simulink model "MBSE_WindowsMIL"  (R2020b)
settings: Solver=VariableStepAuto  StartTime=0.0  StopTime=10.0  RelTol=1e-3
undefined symbols (not defined in the file): sigbuilder_block
libraries: simulink x8
settings Model: Creator=Training  LastModifiedBy=Training

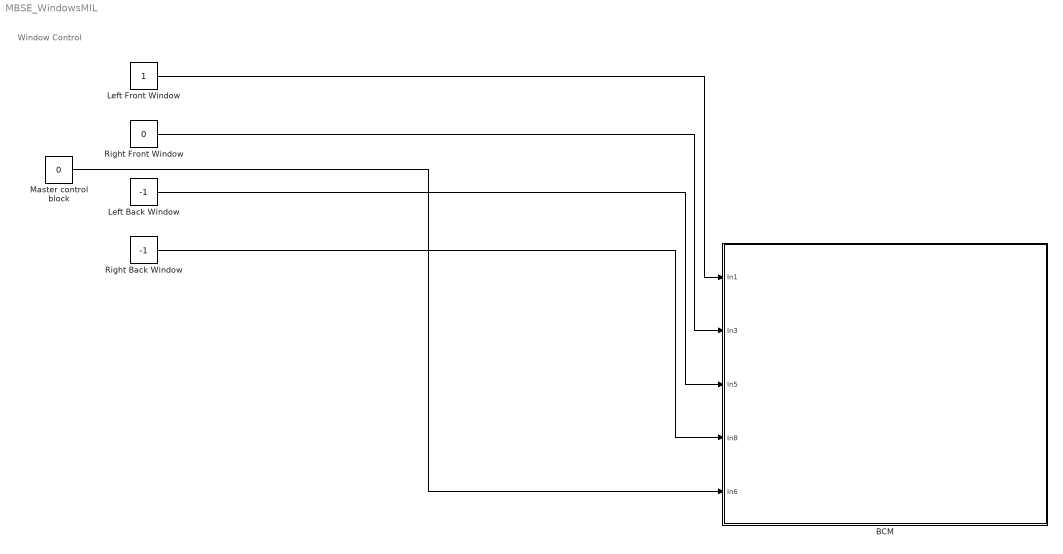
== system MBSE_WindowsMIL ==
  note: Window Control
  BCM : Subsystem
  Left Back Window : Constant  Value=-1
  Left Front Window : Constant
  Master control block : Constant  Value=0
  Right Back Window : Constant  Value=-1
  Right Front Window : Constant  Value=0
  wires:
  Master control block/1 -> BCM/5(In6)
  Right Back Window/1 -> BCM/4(In8)
  Left Back Window/1 -> BCM/3(In5)
  Right Front Window/1 -> BCM/2(In3)
  Left Front Window/1 -> BCM/1(In1)

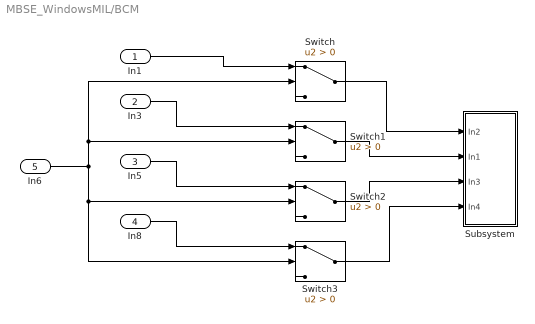
== system MBSE_WindowsMIL/BCM ==
  In1 : Inport
  In3 : Inport  Port=2
  In5 : Inport  Port=3
  In8 : Inport  Port=4
  In6 : Inport  Port=5
  Subsystem : Subsystem
  Switch{,1..3} (4 alike) : Switch  Criteria=u2 > Threshold
  wires:
  In8/1 -> Switch3/1
  In6/1 -> Switch/2, Switch1/2, Switch3/2, Switch2/2
  Switch/1 -> Subsystem/1(In2)
  In3/1 -> Switch1/1
  Switch1/1 -> Subsystem/2(In1)
  In5/1 -> Switch2/1
  Switch3/1 -> Subsystem/4(In4)
  Switch2/1 -> Subsystem/3(In3)
  In1/1 -> Switch/1

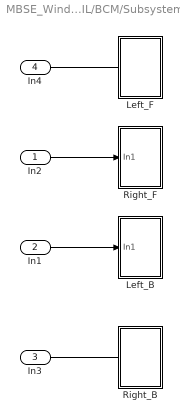
== system MBSE_WindowsMIL/BCM/Subsystem ==
  In2 : Inport
  In1 : Inport  Port=2
  In3 : Inport  Port=3
  In4 : Inport  Port=4
  Left_B : Subsystem
  Left_F : Subsystem
  Right_B : Subsystem
  Right_F : Subsystem
  wires:
  In4/1 -> ?
  In1/1 -> Left_B/1(In1)
  In2/1 -> Right_F/1(In1)
  In3/1 -> ?

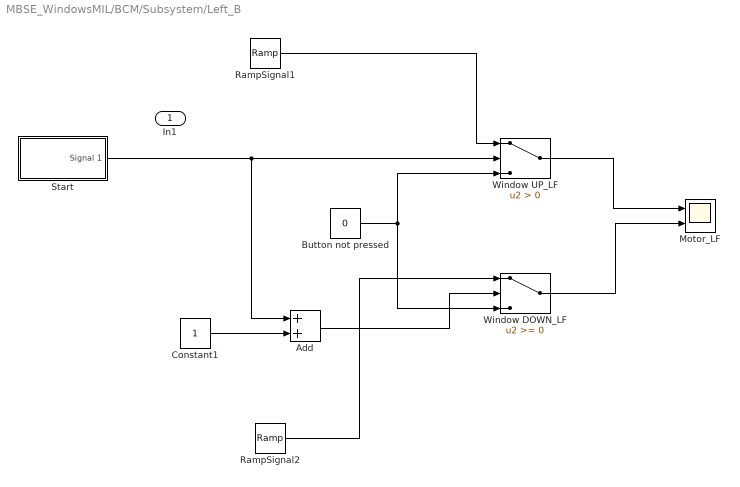
== system MBSE_WindowsMIL/BCM/Subsystem/Left_B ==
  In1 : Inport
  Add : Sum
  Button not pressed : Constant  Value=0
  Constant1 : Constant
  Motor_LF : Scope  NumInputPorts=2
  RampSignal1 : simulink/Sources/Ramp  slope=1  start=0  InitialOutput=0
  RampSignal2 : simulink/Sources/Ramp  slope=1  start=0  InitialOutput=0
  Start : Subsystem  Tag=STV Subsys  LoadFcn=sigbuilder_block('load');  StartFcn=sigbuilder_block('start');  StopFcn=sigbuilder_block('stop');  ClipboardFcn=sigbuilder_block('clipboard');  mask(Sigbuilder block){tuvar=[0:10]}
      mask help: Simulink:masks:SigbuilderBlock_MD
      mask init:
      | if ~strcmp(get_param(bdroot(gcbh),'SimulationStatus'),'stopped') tuvar = sigbuilder_block('maskInit'); end
      settings: CopyFcn=sigbuilder_block('copy');  DeleteFcn=sigbuilder_block('delete');  ModelCloseFcn=sigbuilder_block('modelClose');  PreSaveFcn=sigbuilder_block('preSave');  PauseFcn=sigbuilder_block('pause');  ContinueFcn=sigbuilder_block('continue');  NameChangeFcn=sigbuilder_block('namechange');  OpenFcn=sigbuilder_block('open',[437.6 199.2 550.4 400 ]);  CloseFcn=sigbuilder_block('close');
      mask Display: plot(0, 0, 100, 100,[2, 2, 32, 32, 2], [68, 8, 8, 68, 68],[32, 2], [38, 38], [32, 19, 2],[53, 60, 44], [32, 17, 17, 2],[16, 16, 31, 31]);txt = getActiveGroup(gcbh);text(2, 100, txt,'verticalAlignment', 'top');
  Window DOWN_LF : Switch
  Window UP_LF : Switch  Criteria=u2 > Threshold
  wires:
  Add/1 -> Window DOWN_LF/2
  Button not pressed/1 -> Window UP_LF/3, Window DOWN_LF/3
  Constant1/1 -> Add/2
  RampSignal2/1 -> Window DOWN_LF/1
  Window DOWN_LF/1 -> Motor_LF/2
  Start/1(Signal 1) -> Add/1, Window UP_LF/2
  RampSignal1/1 -> Window UP_LF/1
  Window UP_LF/1 -> Motor_LF/1

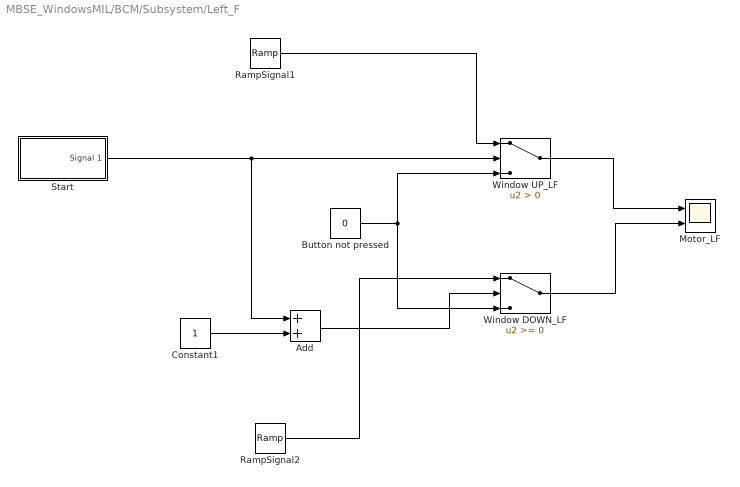
== system MBSE_WindowsMIL/BCM/Subsystem/Left_F ==
  Add : Sum
  Button not pressed : Constant  Value=0
  Constant1 : Constant
  Motor_LF : Scope  NumInputPorts=2
  RampSignal1 : simulink/Sources/Ramp  slope=1  start=0  InitialOutput=0
  RampSignal2 : simulink/Sources/Ramp  slope=1  start=0  InitialOutput=0
  Start : Subsystem  Tag=STV Subsys  LoadFcn=sigbuilder_block('load');  StartFcn=sigbuilder_block('start');  StopFcn=sigbuilder_block('stop');  ClipboardFcn=sigbuilder_block('clipboard');  mask(Sigbuilder block){tuvar=[0:10]}
      mask help: Simulink:masks:SigbuilderBlock_MD
      mask init:
      | if ~strcmp(get_param(bdroot(gcbh),'SimulationStatus'),'stopped') tuvar = sigbuilder_block('maskInit'); end
      settings: CopyFcn=sigbuilder_block('copy');  DeleteFcn=sigbuilder_block('delete');  ModelCloseFcn=sigbuilder_block('modelClose');  PreSaveFcn=sigbuilder_block('preSave');  PauseFcn=sigbuilder_block('pause');  ContinueFcn=sigbuilder_block('continue');  NameChangeFcn=sigbuilder_block('namechange');  OpenFcn=sigbuilder_block('open',[437.6 199.2 550.4 400 ]);  CloseFcn=sigbuilder_block('close');
      mask Display: plot(0, 0, 100, 100,[2, 2, 32, 32, 2], [68, 8, 8, 68, 68],[32, 2], [38, 38], [32, 19, 2],[53, 60, 44], [32, 17, 17, 2],[16, 16, 31, 31]);txt = getActiveGroup(gcbh);text(2, 100, txt,'verticalAlignment', 'top');
  Window DOWN_LF : Switch
  "Window UP_LF " : Switch  Criteria=u2 > Threshold
  wires:
  Add/1 -> Window DOWN_LF/2
  Button not pressed/1 -> "Window UP_LF "/3, Window DOWN_LF/3
  Constant1/1 -> Add/2
  RampSignal2/1 -> Window DOWN_LF/1
  Window DOWN_LF/1 -> Motor_LF/2
  Start/1(Signal 1) -> Add/1, "Window UP_LF "/2
  RampSignal1/1 -> "Window UP_LF "/1
  "Window UP_LF "/1 -> Motor_LF/1

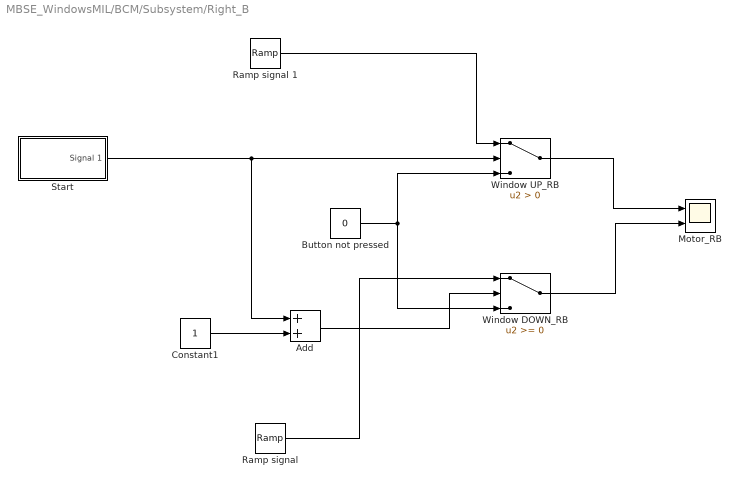
== system MBSE_WindowsMIL/BCM/Subsystem/Right_B ==
  Add : Sum
  Button not pressed : Constant  Value=0
  Constant1 : Constant
  Motor_RB : Scope  NumInputPorts=2
  Ramp signal : simulink/Sources/Ramp  slope=1  start=0  InitialOutput=0
  Ramp signal 1 : simulink/Sources/Ramp  slope=1  start=0  InitialOutput=0
  Start : Subsystem  Tag=STV Subsys  LoadFcn=sigbuilder_block('load');  StartFcn=sigbuilder_block('start');  StopFcn=sigbuilder_block('stop');  ClipboardFcn=sigbuilder_block('clipboard');  mask(Sigbuilder block){tuvar=[0:10]}
      mask help: Simulink:masks:SigbuilderBlock_MD
      mask init:
      | if ~strcmp(get_param(bdroot(gcbh),'SimulationStatus'),'stopped') tuvar = sigbuilder_block('maskInit'); end
      settings: CopyFcn=sigbuilder_block('copy');  DeleteFcn=sigbuilder_block('delete');  ModelCloseFcn=sigbuilder_block('modelClose');  PreSaveFcn=sigbuilder_block('preSave');  PauseFcn=sigbuilder_block('pause');  ContinueFcn=sigbuilder_block('continue');  NameChangeFcn=sigbuilder_block('namechange');  OpenFcn=sigbuilder_block('open',[437.6 199.2 550.4 400 ]);  CloseFcn=sigbuilder_block('close');
      mask Display: plot(0, 0, 100, 100,[2, 2, 32, 32, 2], [68, 8, 8, 68, 68],[32, 2], [38, 38], [32, 19, 2],[53, 60, 44], [32, 17, 17, 2],[16, 16, 31, 31]);txt = getActiveGroup(gcbh);text(2, 100, txt,'verticalAlignment', 'top');
  Window DOWN_RB : Switch
  Window UP_RB : Switch  Criteria=u2 > Threshold
  wires:
  Add/1 -> Window DOWN_RB/2
  Button not pressed/1 -> Window UP_RB/3, Window DOWN_RB/3
  Constant1/1 -> Add/2
  Ramp signal/1 -> Window DOWN_RB/1
  Window DOWN_RB/1 -> Motor_RB/2
  Start/1(Signal 1) -> Add/1, Window UP_RB/2
  Ramp signal 1/1 -> Window UP_RB/1
  Window UP_RB/1 -> Motor_RB/1

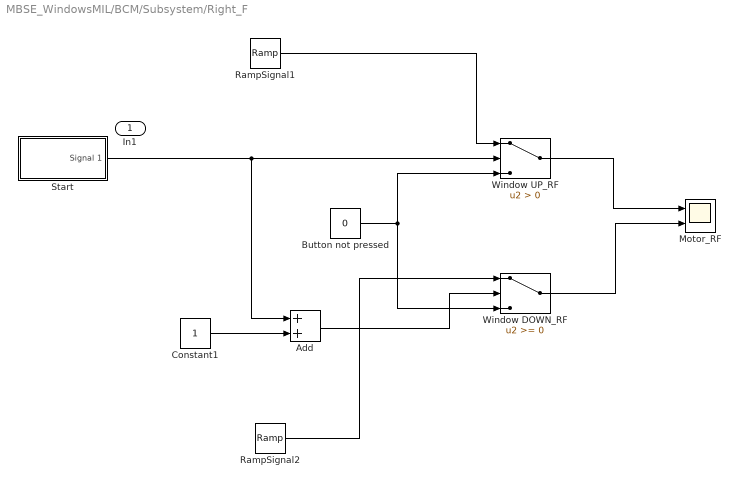
== system MBSE_WindowsMIL/BCM/Subsystem/Right_F ==
  In1 : Inport
  Add : Sum
  Button not pressed : Constant  Value=0
  Constant1 : Constant
  Motor_RF : Scope  NumInputPorts=2
  RampSignal1 : simulink/Sources/Ramp  slope=1  start=0  InitialOutput=0
  RampSignal2 : simulink/Sources/Ramp  slope=1  start=0  InitialOutput=0
  Start : Subsystem  Tag=STV Subsys  LoadFcn=sigbuilder_block('load');  StartFcn=sigbuilder_block('start');  StopFcn=sigbuilder_block('stop');  ClipboardFcn=sigbuilder_block('clipboard');  mask(Sigbuilder block){tuvar=[0:10]}
      mask help: Simulink:masks:SigbuilderBlock_MD
      mask init:
      | if ~strcmp(get_param(bdroot(gcbh),'SimulationStatus'),'stopped') tuvar = sigbuilder_block('maskInit'); end
      settings: CopyFcn=sigbuilder_block('copy');  DeleteFcn=sigbuilder_block('delete');  ModelCloseFcn=sigbuilder_block('modelClose');  PreSaveFcn=sigbuilder_block('preSave');  PauseFcn=sigbuilder_block('pause');  ContinueFcn=sigbuilder_block('continue');  NameChangeFcn=sigbuilder_block('namechange');  OpenFcn=sigbuilder_block('open',[437.6 199.2 550.4 400 ]);  CloseFcn=sigbuilder_block('close');
      mask Display: plot(0, 0, 100, 100,[2, 2, 32, 32, 2], [68, 8, 8, 68, 68],[32, 2], [38, 38], [32, 19, 2],[53, 60, 44], [32, 17, 17, 2],[16, 16, 31, 31]);txt = getActiveGroup(gcbh);text(2, 100, txt,'verticalAlignment', 'top');
  Window DOWN_RF : Switch
  Window UP_RF : Switch  Criteria=u2 > Threshold
  wires:
  Add/1 -> Window DOWN_RF/2
  Button not pressed/1 -> Window UP_RF/3, Window DOWN_RF/3
  Constant1/1 -> Add/2
  RampSignal2/1 -> Window DOWN_RF/1
  Window DOWN_RF/1 -> Motor_RF/2
  Start/1(Signal 1) -> Add/1, Window UP_RF/2
  RampSignal1/1 -> Window UP_RF/1
  Window UP_RF/1 -> Motor_RF/1

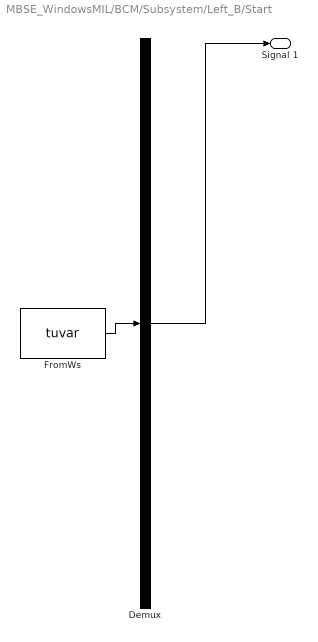
== system MBSE_WindowsMIL/BCM/Subsystem/Left_B/Start ==
  Demux : Demux  Tag=STV Demux  Outputs=1
      settings: DisplayOption=none
  FromWs : FromWorkspace  Tag=STV FromWs  VariableName=tuvar
      SigBuilderData=|
      | common.afterFinalStr = 'Extrapolate'
      | common.sampleTime = 0
      | dataSet.timeRange = [0 10]
      | dataSet.name = 'Group 1'
      | sbobj.Groups.Name = 'Group 1'
      | sbobj.Groups.Signals.Name = 'Signal 1'
      | sbobj.Groups.Signals.XData = [0 4 4 6 6 10]
      | sbobj.Groups.Signals.YData = [0 0 1 1 0 0]
  Signal 1 : Outport  Tag=STV Outport
  wires:
  Demux/1 -> Signal 1/1
  FromWs/1 -> Demux/1

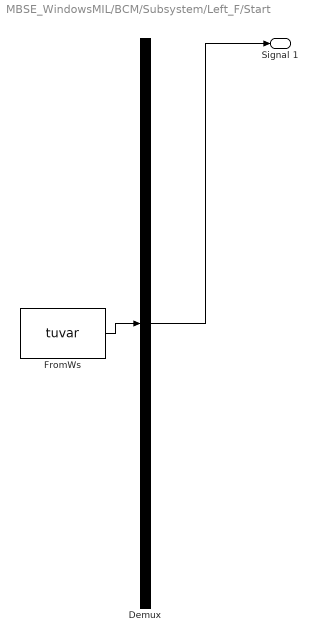
== system MBSE_WindowsMIL/BCM/Subsystem/Left_F/Start ==
  Demux : Demux  Tag=STV Demux  Outputs=1
      settings: DisplayOption=none
  FromWs : FromWorkspace  Tag=STV FromWs  VariableName=tuvar
      SigBuilderData=|
      | common.afterFinalStr = 'Extrapolate'
      | common.sampleTime = 0
      | dataSet.timeRange = [0 10]
      | dataSet.name = 'Group 1'
      | sbobj.Groups.Name = 'Group 1'
      | sbobj.Groups.Signals.Name = 'Signal 1'
      | sbobj.Groups.Signals.XData = [0 4 4 6 6 10]
      | sbobj.Groups.Signals.YData = [0 0 1 1 0 0]
  Signal 1 : Outport  Tag=STV Outport
  wires:
  Demux/1 -> Signal 1/1
  FromWs/1 -> Demux/1

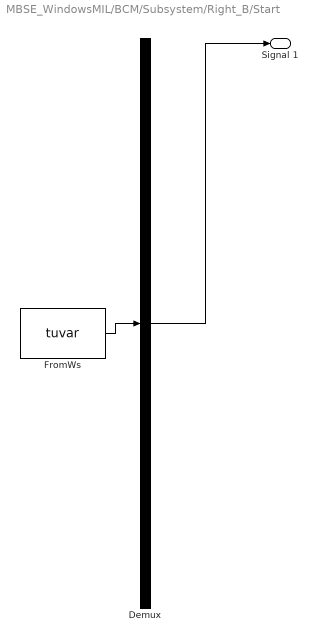
== system MBSE_WindowsMIL/BCM/Subsystem/Right_B/Start ==
  Demux : Demux  Tag=STV Demux  Outputs=1
      settings: DisplayOption=none
  FromWs : FromWorkspace  Tag=STV FromWs  VariableName=tuvar
      SigBuilderData=|
      | common.afterFinalStr = 'Extrapolate'
      | common.sampleTime = 0
      | dataSet.timeRange = [0 10]
      | dataSet.name = 'Group 1'
      | sbobj.Groups.Name = 'Group 1'
      | sbobj.Groups.Signals.Name = 'Signal 1'
      | sbobj.Groups.Signals.XData = [0 4 4 6 6 10]
      | sbobj.Groups.Signals.YData = [0 0 1 1 0 0]
  Signal 1 : Outport  Tag=STV Outport
  wires:
  Demux/1 -> Signal 1/1
  FromWs/1 -> Demux/1

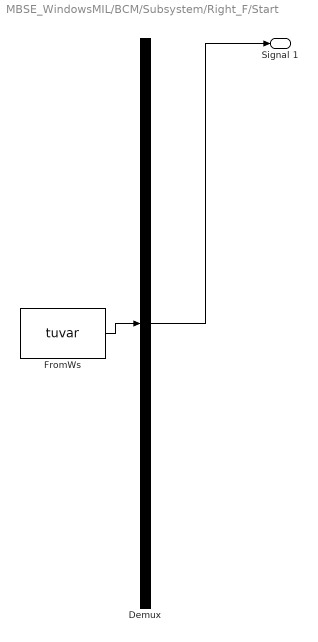
== system MBSE_WindowsMIL/BCM/Subsystem/Right_F/Start ==
  Demux : Demux  Tag=STV Demux  Outputs=1
      settings: DisplayOption=none
  FromWs : FromWorkspace  Tag=STV FromWs  VariableName=tuvar
      SigBuilderData=|
      | common.afterFinalStr = 'Extrapolate'
      | common.sampleTime = 0
      | dataSet.timeRange = [0 10]
      | dataSet.name = 'Group 1'
      | sbobj.Groups.Name = 'Group 1'
      | sbobj.Groups.Signals.Name = 'Signal 1'
      | sbobj.Groups.Signals.XData = [0 4 4 6 6 10]
      | sbobj.Groups.Signals.YData = [0 0 1 1 0 0]
  Signal 1 : Outport  Tag=STV Outport
  wires:
  Demux/1 -> Signal 1/1
  FromWs/1 -> Demux/1
